simulink model "DPWM_VMC_lec21"  (R2017b)
settings: Solver=FixedStepAuto  StartTime=0.0  StopTime=2e-3  FixedStep=Ts  RelTol=1e-3
PostLoadFcn:
  | , if any(exist('dsrtsu_mdlpostloadfcn', 'file') == [2, 3, 6]), try dsrtsu_mdlpostloadfcn('Execute', bdroot); catch fprintf('Error in PostLoadFcn (dsrtsu_mdlpostloadfcn) for model "%s":\n %s\n', bdroot, lasterr); end, end,
  | init_practical_voltage_source;
  | init_parameters;
InitFcn:
  | init_practical_voltage_source;
  | init_parameters;
values from neighbouring files (symbols this model uses):
  DCM_en = 0    [init_parameters.m]
  I0_transient_en = 1    [init_parameters.m]
  ideal_psu_en = 1    [init_parameters.m]
  input_volt_trans_en = 0    [init_parameters.m]
  Kd = 0.5*C    (= 0.0001)    [init_parameters.m]
  Ki = 20000    [init_parameters.m]
  Kp = 30    [init_parameters.m]
  N = 1000    [init_parameters.m]
  Ts = 10e-9    (= 1e-08)    [init_parameters.m]
  Tsw = 2e-6    (= 2e-06)    [init_parameters.m]
  Vff = 1/Vin    (= 0.0833333333333)    [init_parameters.m]
  Vff_en = 1    [init_parameters.m]
  Vin = 12    [init_parameters.m]
  Vmax = 10    [init_parameters.m]
  Vref = 3.3    [init_parameters.m]
  Vref_switch = 1    [init_parameters.m]
libraries: simulink x6
Description:
  | Standard RTI1005 template.
  | Supported MATLAB version:  R2017b.
settings Model: Tag=RTI1005  DSRTSU_INTERNAL_RTI_VER=540  DSRTSU_INTERNAL_RTI_TYPE=rti1005  RTICANMMDATA=struct('GeneralSetupData',struct('modelroot','C:\Projects\Simulink\PE_2\w1\lec7','generalsettings',struct('filesettings',struct('destfolder',struct('Name','RTICANMM_FILES','Check',1),'buildfolder',struct('Name','.','Check',1),'AbsDestfolder',struct('Name','C:\Projects\Simulink\PE_2\w1\lec7\RTICANMM_FILES'),'AbsBuildfolder',struct('Name','C:\Projects\Simulink\PE_2\w1\lec7'))),'options',struct('addpaths',1,'rmpaths',1,'addtrcexclusion',logical(1),'cannavigator',struct('checkmonitoring',0),'show_usrtrc',0,'use_usrtrc',0),'advanced',struct('options',ones(1,100)),'MPSetup',{{}},'RTI',struct('Type','RTI1005','Ver','7.12','Date','02-May-2019'),'modelname','DPWM_VMC_lec21','block','DPWM_VMC_lec21'))  DSRTSU_INTERNAL_RTIFPGA=130  Creator=CA72672  LastModifiedBy=CA72672
settings OptimizationCC: BlockReduction=off  OptimizeBlockIOStorage=off  BufferReuse=off  GlobalBufferReuse=off  ExpressionFolding=off  LocalBlockOutputs=off
settings HardwareCC: ProdBitPerPointer=32  ProdBitPerSizeT=32  ProdBitPerPtrDiffT=32  ProdLargestAtomicInteger=Integer  ProdEndianess=BigEndian  ProdWordSize=32  ProdHWDeviceType=Custom Processor->Custom  TargetIntDivRoundTo=Zero  TargetEndianess=BigEndian  TargetHWDeviceType=Custom Processor->Custom
settings SFSimCC: MATLABDynamicMemAlloc=off
settings RTWCC: SystemTargetFile=rti1005.tlc  MakeCommand=make_rti  TemplateMakefile=rti1005.tmf  Description=dSPACE DS1005 Hardware Platform
settings CodeAppCC: StateflowObjectComments=on
settings STFCustomTargetCC: ParMdlRefBuildCompliant=on  MatFileLogging=on  GRTInterface=off  SystemTargetFile=rti1005.tlc
settings GRTTargetCC: TargetLangStandard=C89/C90 (ANSI)  CompOptLevelCompliant=off  ConcurrentExecutionCompliant=off  CombineOutputUpdateFcns=off  CPPClassGenCompliant=off  UseToolchainInfoCompliant=off
settings ConfigComp: CovMetricSettings=dswe

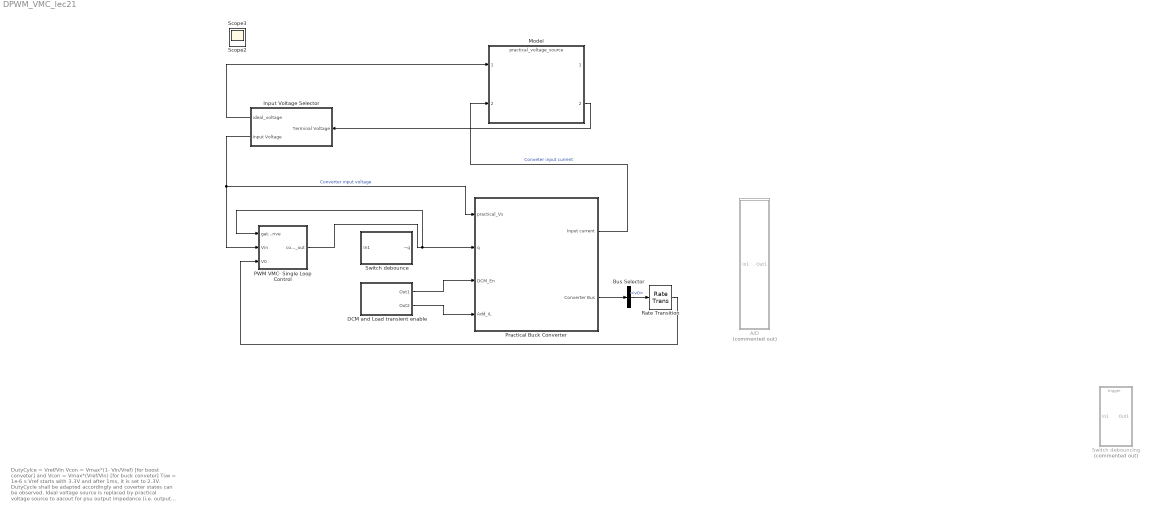
== system DPWM_VMC_lec21 ==
  note: DutyCylce = Vref/Vin
      |
      | Vcon = Vmax*(1- Vin/Vref)	[for boost conveter]
      | and Vcon = Vmax*(Vref/Vin)	[for buck conveter]
      |
      | Tsw = 1e-6 s
      |
      | Vref starts with 3.3V and after 1ms, it is set to 2.3V.
      | DutyCycle shall be adapted accordingly and coverter states can be observed.
      |
      | Ideal voltage source is replaced by practical voltage source to aacout for psu output impedance (i.e. output resistance and finit bandwidt)
      | Input voltage selector lets selection between ideal and practical voltage sources. -->Prameter in the script file: 'ideal_en'
  A/D : Subsystem  Commented=on
  Bus Selector : BusSelector  OutputSignals=v0
  DCM and Load transient enable : Subsystem
  Input Voltage Selector : Subsystem
  Model : ModelReference  ModelNameDialog=practical_voltage_source.slx  SimulationMode=Normal  ModelReferenceVersion=1.13
  PWM VMC- Single Loop Control : Subsystem
  Practical Buck Converter : Subsystem
  Rate Transition : RateTransition  OutPortSampleTime=Tsw
  Switch debounce : Subsystem
  Switch debouncing : Subsystem  Commented=on  TreatAsAtomicUnit=on
  Scope2 : Scope
  Scope3 : Scope
  wires:
  DCM and Load transient enable/1(Out1) -> Practical Buck Converter/3(DCM_En)
  DCM and Load transient enable/2(Out2) -> Practical Buck Converter/4(Add_iL)
  Practical Buck Converter/1(Input current) -> Model/2  "Conveter input current"
  Input Voltage Selector/2(Input Voltage) -> Practical Buck Converter/1(practical_Vs), PWM VMC- Single Loop Control/2(Vin)  "Converter input voltage"
  Input Voltage Selector/1(ideal_voltage) -> Model/1
  Model/2 -> Input Voltage Selector/1(Terminal Voltage)
  PWM VMC- Single Loop Control/1(comp_out) -> PWM VMC- Single Loop Control/1(gate_drive), Practical Buck Converter/2(q)
  Practical Buck Converter/2(Converter Bus) -> Bus Selector/1
  Rate Transition/1 -> PWM VMC- Single Loop Control/3(V0)
  Bus Selector/1 -> Rate Transition/1  "<v0>"

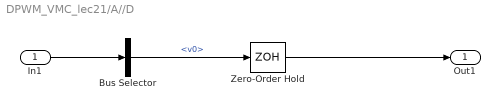
== system DPWM_VMC_lec21/A//D ==
  In1 : Inport
  Bus Selector : BusSelector  OutputSignals=v0
  "Zero-Order Hold " : ZeroOrderHold  SampleTime=Tsw
  Out1 : Outport
  wires:
  In1/1 -> Bus Selector/1
  Bus Selector/1 -> "Zero-Order Hold "/1  "<v0>"
  "Zero-Order Hold "/1 -> Out1/1

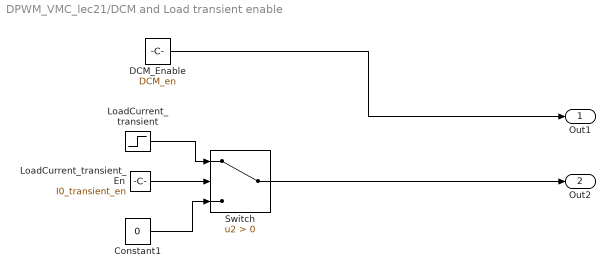
== system DPWM_VMC_lec21/DCM and Load transient enable ==
  Constant1 : Constant  Value=0
  DCM_Enable : Constant  Value=DCM_en  OutDataTypeStr=boolean
  LoadCurrent_transient : Step  Time=1.0e-3  After=20  SampleTime=Ts
  LoadCurrent_transient_En : Constant  Value=I0_transient_en  OutDataTypeStr=boolean
  Switch : Switch  Criteria=u2 > Threshold
  Out1 : Outport
  Out2 : Outport  Port=2
  wires:
  Switch/1 -> Out2/1
  DCM_Enable/1 -> Out1/1
  Constant1/1 -> Switch/3
  LoadCurrent_transient_En/1 -> Switch/2
  LoadCurrent_transient/1 -> Switch/1

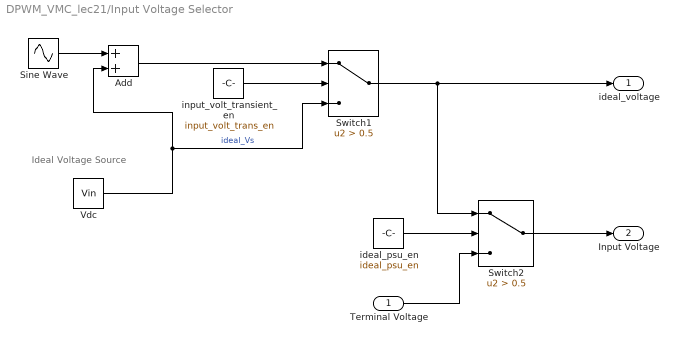
== system DPWM_VMC_lec21/Input Voltage Selector ==
  note: Ideal Voltage Source
  Terminal Voltage : Inport
  Add : Sum
  Sine Wave : Sin  Amplitude=2  Frequency=2*pi*1e3  SampleTime=0
  Switch1 : Switch  Criteria=u2 > Threshold  Threshold=0.5
  Switch2 : Switch  Criteria=u2 > Threshold  Threshold=0.5
  Vdc : Constant  Value=Vin
  ideal_psu_en : Constant  Value=ideal_psu_en
  input_volt_transient_en : Constant  Value=input_volt_trans_en
  ideal_voltage : Outport
  Input Voltage : Outport  Port=2
  wires:
  Vdc/1 -> Add/2, Switch1/3  "ideal_Vs"
  Add/1 -> Switch1/1
  input_volt_transient_en/1 -> Switch1/2
  Switch1/1 -> Switch2/1, ideal_voltage/1
  Sine Wave/1 -> Add/1
  Switch2/1 -> Input Voltage/1
  ideal_psu_en/1 -> Switch2/2
  Terminal Voltage/1 -> Switch2/3

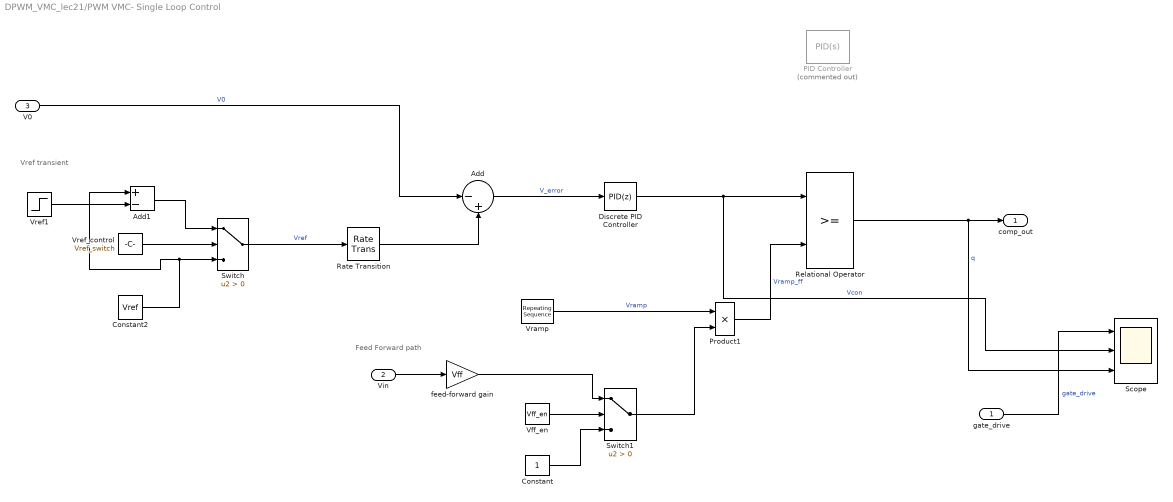
== system DPWM_VMC_lec21/PWM VMC- Single Loop Control ==
  note: Vref transient
  note: Feed Forward path
  gate_drive : Inport
  Vin : Inport  Port=2
  V0 : Inport  Port=3
  Add : Sum  Inputs=|-+
  Add1 : Sum  Inputs=+-
  Constant : Constant
  Constant2 : Constant  Value=Vref
  Discrete PID Controller : simulink/Continuous/PID Controller  Controller=PID  TimeDomain=Discrete-time  SampleTime=-1  IntegratorMethod=Forward Euler  FilterMethod=Forward Euler  Form=Parallel  UseFilter=off  ControllerParametersSource=internal  P=Kp  I=Ki  D=Kd  N=N  InitialConditionSource=internal  InitialConditionForIntegrator=0  InitialConditionForFilter=0  ExternalReset=none  LimitOutput=off  UpperSaturationLimit=inf  LowerSaturationLimit=-inf  LinearizeAsGain=off  AntiWindupMode=none  Kb=1  TrackingMode=off  Kt=1  PParamMin=[]  PParamMax=[]  IParamMin=[]  IParamMax=[]  DParamMin=[]  DParamMax=[]  NParamMin=[]  NParamMax=[]  KbParamMin=[]  KbParamMax=[]  KtParamMin=[]  KtParamMax=[]  POutMin=[]  POutMax=[]  IOutMin=[]  IOutMax=[]  DOutMin=[]  DOutMax=[]  NOutMin=[]  NOutMax=[]  KbOutMin=[]  KbOutMax=[]  KtOutMin=[]  KtOutMax=[]  IntegratorOutMin=[]  IntegratorOutMax=[]  FilterOutMin=[]  FilterOutMax=[]  SumOutMin=[]  SumOutMax=[]  SumI1OutMin=[]  SumI1OutMax=[]  SumI2OutMin=[]  SumI2OutMax=[]  SumI3OutMin=[]  SumI3OutMax=[]  SumDOutMin=[]  SumDOutMax=[]  SaturationOutMin=[]  SaturationOutMax=[]  IntegratorContinuousStateAttributes=''  IntegratorStateMustResolveToSignalObject=off  IntegratorRTWStateStorageClass=Auto  FilterContinuousStateAttributes=''  FilterStateMustResolveToSignalObject=off  FilterRTWStateStorageClass=Auto  DifferentiatorICPrevScaledInput=0  DifferentiatorOutMin=[]  DifferentiatorOutMax=[]  InitialConditionSetting=State (most efficient)  FilterDiffOutCoefMin=[]  FilterDiffOutCoefMax=[]  SumDenOutMin=[]  SumDenOutMax=[]  SumNumOutMin=[]  SumNumOutMax=[]  ReciprocalOutMin=[]  ReciprocalOutMax=[]  DivideOutMin=[]  DivideOutMax=[]  TunerSelectOption=Transfer Function Based (PID Tuner App)
  PID Controller : simulink/Continuous/PID Controller  Commented=on  Controller=PID  TimeDomain=Continuous-time  SampleTime=-1  IntegratorMethod=Forward Euler  FilterMethod=Forward Euler  Form=Parallel  UseFilter=on  ControllerParametersSource=internal  P=Kp  I=Ki  D=Kd  N=N  InitialConditionSource=internal  InitialConditionForIntegrator=0  InitialConditionForFilter=0  ExternalReset=none  LimitOutput=off  UpperSaturationLimit=inf  LowerSaturationLimit=-inf  LinearizeAsGain=on  AntiWindupMode=none  Kb=1  TrackingMode=off  Kt=1  PParamMin=[]  PParamMax=[]  IParamMin=[]  IParamMax=[]  DParamMin=[]  DParamMax=[]  NParamMin=[]  NParamMax=[]  KbParamMin=[]  KbParamMax=[]  KtParamMin=[]  KtParamMax=[]  POutMin=[]  POutMax=[]  IOutMin=[]  IOutMax=[]  DOutMin=[]  DOutMax=[]  NOutMin=[]  NOutMax=[]  KbOutMin=[]  KbOutMax=[]  KtOutMin=[]  KtOutMax=[]  IntegratorOutMin=[]  IntegratorOutMax=[]  FilterOutMin=[]  FilterOutMax=[]  SumOutMin=[]  SumOutMax=[]  SumI1OutMin=[]  SumI1OutMax=[]  SumI2OutMin=[]  SumI2OutMax=[]  SumI3OutMin=[]  SumI3OutMax=[]  SumDOutMin=[]  SumDOutMax=[]  SaturationOutMin=[]  SaturationOutMax=[]  IntegratorContinuousStateAttributes=''  IntegratorStateMustResolveToSignalObject=off  IntegratorRTWStateStorageClass=Auto  FilterContinuousStateAttributes=''  FilterStateMustResolveToSignalObject=off  FilterRTWStateStorageClass=Auto  DifferentiatorICPrevScaledInput=0  DifferentiatorOutMin=[]  DifferentiatorOutMax=[]  InitialConditionSetting=State (most efficient)  FilterDiffOutCoefMin=[]  FilterDiffOutCoefMax=[]  SumDenOutMin=[]  SumDenOutMax=[]  SumNumOutMin=[]  SumNumOutMax=[]  ReciprocalOutMin=[]  ReciprocalOutMax=[]  DivideOutMin=[]  DivideOutMax=[]  TunerSelectOption=Transfer Function Based (PID Tuner App)
  Product1 : Product
  Rate Transition : RateTransition  OutPortSampleTime=Tsw
  Relational Operator : RelationalOperator  OutDataTypeStr=boolean  RndMeth=Simplest
  Scope : Scope  NumInputPorts=3
  Switch : Switch  Criteria=u2 > Threshold
  Switch1 : Switch  Criteria=u2 > Threshold
  Vff_en : Constant  Value=Vff_en
  Vramp : simulink/Sources/Repeating Sequence  rep_seq_t=[0 Tsw]  rep_seq_y=[0 Vmax]
  Vref1 : Step  Time=1.25e-3  After=0.5  SampleTime=Ts
  Vref_control : Constant  Value=Vref_switch
  feed-forward gain : Gain  Gain=Vff
  comp_out : Outport
  wires:
  Discrete PID Controller/1 -> Scope/2, Relational Operator/1  "Vcon"
  Add/1 -> Discrete PID Controller/1  "V_error"
  Switch/1 -> Rate Transition/1  "Vref"
  Vff_en/1 -> Switch1/2
  Vin/1 -> feed-forward gain/1
  Vramp/1 -> Product1/1  "Vramp"
  Constant/1 -> Switch1/3
  feed-forward gain/1 -> Switch1/1
  Relational Operator/1 -> Scope/3, comp_out/1  "q"
  Product1/1 -> Relational Operator/2  "Vramp_ff"
  gate_drive/1 -> Scope/1  "gate_drive"
  Constant2/1 -> Add1/1, Switch/3
  Add1/1 -> Switch/1
  Vref_control/1 -> Switch/2
  Vref1/1 -> Add1/2
  V0/1 -> Add/1  "V0"
  Switch1/1 -> Product1/2
  Rate Transition/1 -> Add/2

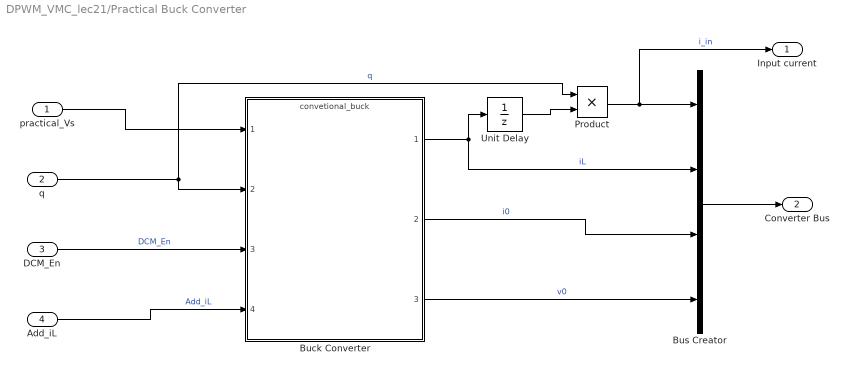
== system DPWM_VMC_lec21/Practical Buck Converter ==
  practical_Vs : Inport
  q : Inport  Port=2
  DCM_En : Inport  Port=3
  Add_iL : Inport  Port=4
  Buck Converter : ModelReference  ModelNameDialog=convetional_buck.slx  SimulationMode=Normal  ModelReferenceVersion=1.37
  Bus Creator : BusCreator  Inputs=4
  Product : Product
  Unit Delay : UnitDelay  SampleTime=-1
  Input current : Outport
  Converter Bus : Outport  Port=2
  wires:
  practical_Vs/1 -> Buck Converter/1
  DCM_En/1 -> Buck Converter/3  "DCM_En"
  Add_iL/1 -> Buck Converter/4  "Add_iL"
  Buck Converter/2 -> Bus Creator/3  "i0"
  Buck Converter/1 -> Bus Creator/2, Unit Delay/1  "iL"
  Buck Converter/3 -> Bus Creator/4  "v0"
  q/1 -> Buck Converter/2, Product/1  "q"
  Product/1 -> Input current/1, Bus Creator/1  "i_in"
  Unit Delay/1 -> Product/2
  Bus Creator/1 -> Converter Bus/1

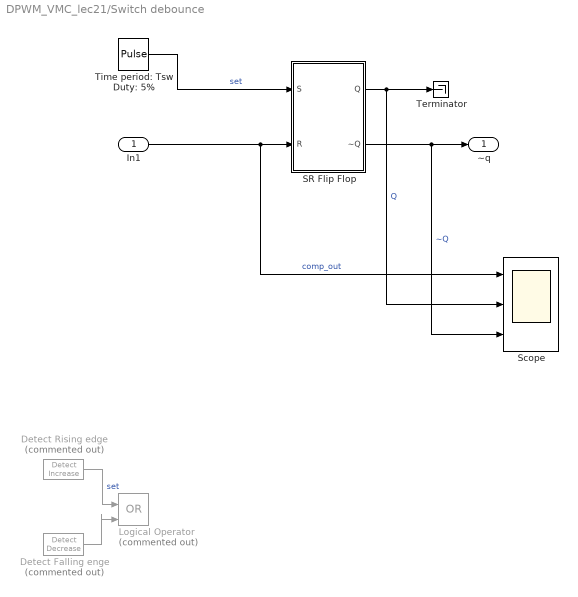
== system DPWM_VMC_lec21/Switch debounce ==
  In1 : Inport
  Detect Falling enge : simulink/Logic and Bit Operations/Detect Decrease  Commented=on  vinit=0.0  OutDataTypeStr=boolean
  Detect Rising edge : simulink/Logic and Bit Operations/Detect Increase  Commented=on  vinit=0.0  OutDataTypeStr=boolean
  Logical Operator : Logic  Commented=on  Operator=OR  IconShape=distinctive  AllPortsSameDT=off  OutDataTypeStr=boolean
  SR Flip Flop : Subsystem
  Scope : Scope  NumInputPorts=3
  Terminator : Terminator
  Time period: Tsw Duty: 5% : DiscretePulseGenerator  PulseType=Time based  Period=Tsw  PulseWidth=5
  ~q : Outport
  wires:
  SR Flip Flop/2(~Q) -> Scope/3, ~q/1  "~Q"
  SR Flip Flop/1(Q) -> Scope/2, Terminator/1  "Q"
  In1/1 -> Scope/1, SR Flip Flop/2(R)  "comp_out"
  Detect Falling enge/1 -> Logical Operator/2
  Detect Rising edge/1 -> Logical Operator/1  "set"
  Time period: Tsw Duty: 5%/1 -> SR Flip Flop/1(S)  "set"

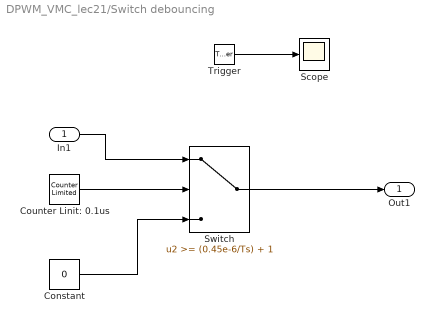
== system DPWM_VMC_lec21/Switch debouncing ==
  In1 : Inport
  Trigger : TriggerPort  VariantControl=Variant  ShowOutputPort=on  PortDimensions=1
  Constant : Constant  Value=0
  Counter Linit: 0.1us : simulink/Sources/Counter Limited  uplimit=(0.45e-6/Ts) + 1  tsamp=-1
  Scope : Scope
  Switch : Switch  Threshold=(0.45e-6/Ts) + 1
  Out1 : Outport
  wires:
  In1/1 -> Switch/1
  Switch/1 -> Out1/1
  Counter Linit: 0.1us/1 -> Switch/2
  Constant/1 -> Switch/3
  Trigger/1 -> Scope/1

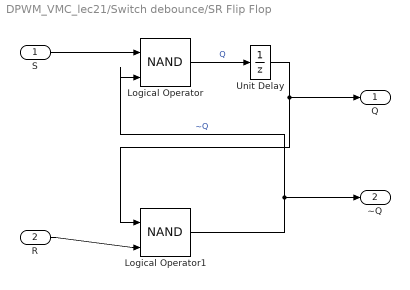
== system DPWM_VMC_lec21/Switch debounce/SR Flip Flop ==
  S : Inport
  R : Inport  Port=2
  Logical Operator : Logic  Operator=NAND  IconShape=distinctive  AllPortsSameDT=off  OutDataTypeStr=boolean
  Logical Operator1 : Logic  Operator=NAND  IconShape=distinctive  AllPortsSameDT=off  OutDataTypeStr=boolean
  Unit Delay : UnitDelay  SampleTime=-1
  Q : Outport
  ~Q : Outport  Port=2
  wires:
  S/1 -> Logical Operator/1
  R/1 -> Logical Operator1/2
  Logical Operator/1 -> Unit Delay/1  "Q"
  Logical Operator1/1 -> ~Q/1, Logical Operator/2  "~Q"
  Unit Delay/1 -> Q/1, Logical Operator1/1
